simulink model "Loadflow2_1_source"  (R2016b)
settings: Solver=ode1  StartTime=0.0  StopTime=10.0  FixedStep=Time_Step  MaxStep=50e-6  RelTol=1e-3
undefined symbols (not defined in the file): fb, L, R, Theta0, Time_Step, Vm_RMS, Vn
libraries: powerlib x12, powerlib_meascontrol x2
settings Model: Creator=Frederic_Colas  LastModifiedBy=Frederic_Colas
settings DataIOCC: ReturnWorkspaceOutputs=on
settings SFSimCC: SimUseLocalCustomCode=on
settings RTWCC: RTWUseLocalCustomCode=on

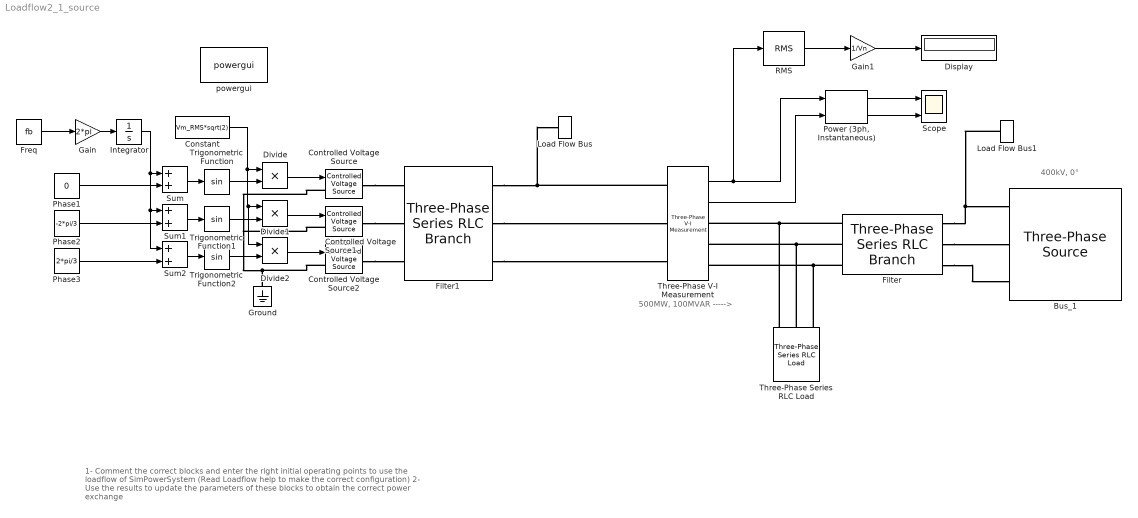
== system Loadflow2_1_source ==
  note: 500MW, 100MVAR
      | ----->
  note: 400kV, 0°
  note: 1- Comment the correct blocks and enter the right initial operating points to use the loadflow of SimPowerSystem (Read Loadflow help to make the correct configuration)
      |
      | 2- Use the results to update the parameters of these blocks to obtain the correct power exchange
  Bus_1 : powerlib/Electrical Sources/Three-Phase Source  InternalConnection=Yg  VoltagePhases=off  Voltage=(400000)*1  PhaseAngle=0  Voltage_phases=[25e3 25e3 25e3]/sqrt(3)  PhaseAngles_phases=[0 -120 +120]  Frequency=fb  NonIdealSource=off  SpecifyImpedance=off  Resistance=0.8929  Inductance=16.58e-3  ShortCircuitLevel=100e6  BaseVoltage=25e3  XRratio=7  BusType=swing  Pref=10e3  Qref=0  Prefabc=[10e3, 10e3, 10e3]  Qrefabc=[0, 0, 0]  Qmin=-inf  Qmax=inf
  Constant : Constant  Value=Vm_RMS*sqrt(2)
  Controlled Voltage Source : powerlib/Electrical Sources/Controlled Voltage Source  Initialize=on  Source_Type=AC  Amplitude=Vm_RMS*sqrt(2)  Phase=Theta0*pi/180  Frequency=fb  Measurements=None
  Controlled Voltage Source1 : powerlib/Electrical Sources/Controlled Voltage Source  Initialize=on  Source_Type=AC  Amplitude=Vm_RMS*sqrt(2)  Phase=Theta0*pi/180-2*pi/3  Frequency=fb  Measurements=None
  Controlled Voltage Source2 : powerlib/Electrical Sources/Controlled Voltage Source  Initialize=on  Source_Type=AC  Amplitude=Vm_RMS*sqrt(2)  Phase=Theta0*pi/180-4*pi/3  Frequency=fb  Measurements=None
  Display : Display
  Divide : Product  Inputs=**
  Divide1 : Product  Inputs=**
  Divide2 : Product  Inputs=**
  Filter : powerlib/Elements/Three-Phase Series RLC Branch  LConnTagsString=A|B|C  RConnTagsString=A|B|C  BranchType=RL  Resistance=0.2546*5  Inductance=0.0187*5  Capacitance=1e-6  Measurements=None
  Filter1 : powerlib/Elements/Three-Phase Series RLC Branch  LConnTagsString=A|B|C  RConnTagsString=A|B|C  BranchType=RL  Resistance=R  Inductance=L  Capacitance=1e-6  Measurements=None
  Freq : Constant  Value=fb
  Gain : Gain  Gain=2*pi
  Gain1 : Gain  Gain=1/Vn
  Ground : powerlib/Elements/Ground  LConnTagsString=a
  Integrator : Integrator  InitialCondition=Theta0*pi/180
  Load Flow Bus : powerlib/Measurements/Load Flow Bus  LConnTagsString=a  Phases=single  Connectors=on one side  ID=BUS_2  Vbase=Un  Vref=1  Vangle=0  VLF=0.9827  VLFb=1  VLFc=1  angleLF=0.2265  angleLFb=0  angleLFc=0
  Load Flow Bus1 : powerlib/Measurements/Load Flow Bus  LConnTagsString=a  Phases=single  Connectors=on one side  ID=BUS_1  Vbase=Un  Vref=1  Vangle=0  VLF=1  VLFb=1  VLFc=1  angleLF=0  angleLFb=0  angleLFc=0
  Phase1 : Constant  Value=0
  Phase2 : Constant  Value=-2*pi/3
  Phase3 : Constant  Value=2*pi/3
  "Power (3ph, Instantaneous)" : powerlib_meascontrol/Measurements/Power (3ph, Instantaneous)
  RMS : powerlib_meascontrol/Measurements/RMS  TrueRMS=on  Freq=fb  RMSInit=Vn  Ts=0
  Scope : Scope  NumInputPorts=2
  Sum : Sum
  Sum1 : Sum
  Sum2 : Sum
  Three-Phase Series RLC Load : powerlib/Elements/Three-Phase Series RLC Load  LConnTagsString=A|B|C  Configuration=Y (grounded)  NominalVoltage=400e3  Vabc=[1e3 1e3 1e3]  Vabcp=[1e3 1e3 1e3]  NominalFrequency=50  UnbalancedPower=off  ActivePower=500e6  InductivePower=200e6  CapacitivePower=0  Pabc=[10e3 9e3 11e3]  QLabc=[100 90 110]  QCabc=[100 90 110]  Pabcp=[10e3 9e3 11e3]  QLabcp=[100 90 110]  QCabcp=[100 90 110]  Measurements=None  LoadType=constant Z
  Three-Phase V-I Measurement : powerlib/Measurements/Three-Phase V-I Measurement  VoltageMeasurement=phase-to-ground  SetLabelV=off  LabelV=Vabc  Vpu=off  VpuLL=off  CurrentMeasurement=yes  SetLabelI=off  LabelI=Iabc  Ipu=off  Pbase=100e6  Vbase=500e3  OutputType=Complex  PhasorSimulation=off  PSBequivalent=0
  Trigonometric Function : Trigonometry
  Trigonometric Function1 : Trigonometry
  Trigonometric Function2 : Trigonometry
  powergui : powerlib/powergui  Priority=1  SimulationMode=Discrete  SampleTime=Time_Step  frequency=60  Iterations=50  frequencyindice=50  Pbase=1000000000  ErrMax=1e-06  UnitsV=kV  UnitsW=MW  buscounter=0  FunctionMessages=off  echomessages=off  EnableUseOfTLC=off  CurrentSourceSwitches=off  DisableSnubberDevices=off  DisableRonSwitches=off  DisableVfSwitches=off  DisplayEquations=off  AutomaticDiscreteSolvers=off  SolverType=Tustin/Backward Euler (TBE)  Interpol=off  ExternalGateDelay=off  methode=off  Ts=100  x0status=blocks  SPID=on  SwTol=0  HookPort=off  NonlinearTolerance=1e-4  nMaxIteration=100  ContinueOnMaxIteration=off  RestoreLinks=warning  ResistiveCurrentMeasurement=off  Frange=[0:2:500]  Ylog=off  Xlog=on  ShowGrid=off  save=off  variable=ZData  structure=0  ZoomFFT=off  StartTime=0.0  cycles=1  DisplayStyle=1  fundamental=60  FreqAxis=off  MaxFrequency=1000  frequencyindicesteady=1  RmsSteady=1  display=off
  wires:
  Three-Phase V-I Measurement/1 -> RMS/1, "Power (3ph, Instantaneous)"/1
  Three-Phase V-I Measurement/2 -> "Power (3ph, Instantaneous)"/2
  "Power (3ph, Instantaneous)"/1 -> Scope/1
  "Power (3ph, Instantaneous)"/2 -> Scope/2
  Constant/1 -> Divide2/1, Divide1/1, Divide/1
  Integrator/1 -> Sum2/1, Sum1/1, Sum/1
  Freq/1 -> Gain/1
  Phase3/1 -> Sum2/2
  Gain/1 -> Integrator/1
  Divide2/1 -> Controlled Voltage Source2/1
  Sum/1 -> Trigonometric Function/1
  Phase2/1 -> Sum1/2
  Trigonometric Function/1 -> Divide/2
  Sum1/1 -> Trigonometric Function1/1
  Divide/1 -> Controlled Voltage Source/1
  Sum2/1 -> Trigonometric Function2/1
  Trigonometric Function2/1 -> Divide2/2
  Trigonometric Function1/1 -> Divide1/2
  Divide1/1 -> Controlled Voltage Source1/1
  Phase1/1 -> Sum/2
  RMS/1 -> Gain1/1
  Gain1/1 -> Display/1
  connections:
  Three-Phase V-I Measurement/LConn1 -- Filter1/RConn1 -- Load Flow Bus/LConn1
  Filter/LConn1 -- Three-Phase Series RLC Load/LConn1 -- Three-Phase V-I Measurement/RConn1
  Filter/LConn2 -- Three-Phase Series RLC Load/LConn2 -- Three-Phase V-I Measurement/RConn2
  Filter/LConn3 -- Three-Phase Series RLC Load/LConn3 -- Three-Phase V-I Measurement/RConn3
  Filter/RConn2 -- Bus_1/RConn2
  Load Flow Bus1/LConn1 -- Filter/RConn1 -- Bus_1/RConn1
  Filter/RConn3 -- Bus_1/RConn3
  Filter1/RConn2 -- Three-Phase V-I Measurement/LConn2
  Filter1/RConn3 -- Three-Phase V-I Measurement/LConn3
  Controlled Voltage Source2/LConn1 -- Ground/LConn1 -- Controlled Voltage Source/LConn1 -- Controlled Voltage Source1/LConn1
  Controlled Voltage Source2/RConn1 -- Filter1/LConn3
  Controlled Voltage Source/RConn1 -- Filter1/LConn1
  Controlled Voltage Source1/RConn1 -- Filter1/LConn2
